simulink model "mcb_microchip_pmsm_posCtrl_SAME70"  (R2022a)
settings: Solver=FixedStepDiscrete  StartTime=0.0  StopTime=6  RelTol=1e-3  EnableMultiTasking=on
InitFcn:
  | mcb_microchip_pmsm_posCtrl_SAME70_data;
values from neighbouring files (symbols this model uses):
  PI_params = mcb.internal.SetControllerParameters(pmsm,inverter,PU_System,T_pwm,2*Ts,Ts_speed)    [mcb_microchip_pmsm_posCtrl_SAME70_data.m]
  PosCtrlSpeedLimit = 0.1    [mcb_microchip_pmsm_posCtrl_SAME70_data.m]
  PU_System = mcb_SetPUSystem(pmsm,inverter)    [mcb_microchip_pmsm_posCtrl_SAME70_data.m]
  PWM_frequency = 20e3    (= 20000)    [mcb_microchip_pmsm_posCtrl_SAME70_data.m]
  Ts = T_pwm    (= 5e-05)    [mcb_microchip_pmsm_posCtrl_SAME70_data.m]
  Ts_motor = T_pwm/2    (= 2.5e-05)    [mcb_microchip_pmsm_posCtrl_SAME70_data.m]
  Ts_simulink = T_pwm/2    (= 2.5e-05)    [mcb_microchip_pmsm_posCtrl_SAME70_data.m]
  Ts_speed = 2 * Ts    (= 0.0001)    [mcb_microchip_pmsm_posCtrl_SAME70_data.m]
undefined symbols (not defined in the file or in its folder): A24, AD10, AD7, inverter, LQFP144, MaxPer, ms, ns, PA0, PA1, PA10, PA11, PA12, PA13, PA16, PA18, PA9, PB0, PD18, PD19, PD24, PD25, PD26, Pin, pmsm, Resol, SAME70Q21B, Timer, Unsigned
libraries: MCHP_Blockset x13, simulink x13, mcbcontrolslib x8, slpidlib x3, mcbpositiondecoderlib x3, mcbplantlib x1, autolibpmsmexterior x1
(part 3 of 4)

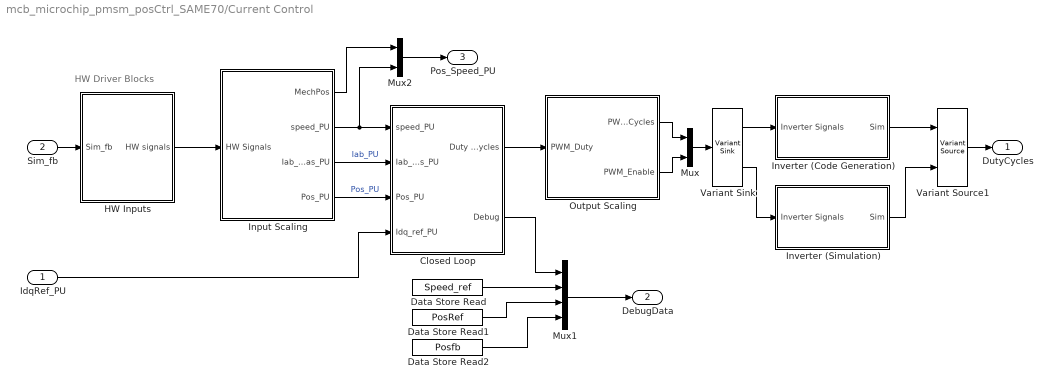
== system mcb_microchip_pmsm_posCtrl_SAME70/Current Control ==
  note: HW Driver Blocks
  IdqRef_PU : Inport
  Sim_fb : Inport  Port=2
  Closed Loop : Subsystem
  Data Store Read : DataStoreRead  DataStoreName=Speed_ref  IndexOptions=Index vector (dialog)  Indices=1  OutputSizes=1
  Data Store Read1 : DataStoreRead  DataStoreName=PosRef  IndexOptions=Index vector (dialog)  Indices=1  OutputSizes=1
  Data Store Read2 : DataStoreRead  DataStoreName=Posfb  IndexOptions=Index vector (dialog)  Indices=1  OutputSizes=1
  HW Inputs : Subsystem  Variant=on  VariantControlMode=sim codegen switching
  Input Scaling : Subsystem
  Inverter (Code Generation) : Subsystem
  Inverter (Simulation) : Subsystem
  Mux : Mux  Inputs=2
  Mux1 : Mux
  Mux2 : Mux  Inputs=2
  Output Scaling : Subsystem
  Variant Sink : VariantSink  VariantControlMode=sim codegen switching
  Variant Source1 : VariantSource  VariantControlMode=sim codegen switching
  DutyCycles : Outport  InitialOutput=0  VectorParamsAs1DForOutWhenUnconnected=off
  DebugData : Outport  Port=2
  Pos_Speed_PU : Outport  Port=3  InitialOutput=0  VectorParamsAs1DForOutWhenUnconnected=off
  wires:
  Closed Loop/1(Duty Cycles) -> Output Scaling/1(PWM_Duty)
  IdqRef_PU/1 -> Closed Loop/4(Idq_ref_PU)
  Output Scaling/2(PWM_Enable) -> Mux/2
  Input Scaling/2(speed_PU) -> Mux2/2, Closed Loop/1(speed_PU)
  Sim_fb/1 -> HW Inputs/1(Sim_fb)
  Input Scaling/3(Iab_meas_PU) -> Closed Loop/2(Iab_meas_PU)  "Iab_PU"
  Input Scaling/4(Pos_PU) -> Closed Loop/3(Pos_PU)  "Pos_PU"
  Variant Source1/1 -> DutyCycles/1
  Output Scaling/1(PWM_Duty_Cycles) -> Mux/1
  Variant Sink/2 -> Inverter (Simulation)/1(Inverter Signals)
  Inverter (Code Generation)/1(Sim) -> Variant Source1/1
  Inverter (Simulation)/1(Sim) -> Variant Source1/2
  Variant Sink/1 -> Inverter (Code Generation)/1(Inverter Signals)
  Mux/1 -> Variant Sink/1
  HW Inputs/1(HW signals) -> Input Scaling/1(HW Signals)
  Mux1/1 -> DebugData/1
  Closed Loop/2(Debug) -> Mux1/1
  Data Store Read/1 -> Mux1/2
  Mux2/1 -> Pos_Speed_PU/1
  Input Scaling/1(MechPos) -> Mux2/1
  Data Store Read1/1 -> Mux1/3
  Data Store Read2/1 -> Mux1/4

== system mcb_microchip_pmsm_posCtrl_SAME70/Heartbeat LED ==
  note: Heartbeat LED 1HZ
  Code generation : Subsystem
  RED_LED : Constant  OutDataTypeStr=uint16  SampleTime=0.25
  Simulation : Subsystem
  Variant Sink : VariantSink
  wires:
  RED_LED/1 -> Variant Sink/1
  Variant Sink/1 -> Code generation/1(In1)
  Variant Sink/2 -> Simulation/1(In1)

== system mcb_microchip_pmsm_posCtrl_SAME70/Inverter and Motor ==
  Duty_Cycles : Inport
  Plant Model : Subsystem  Variant=on  VariantControlMode=sim codegen switching  VariantControl=Variant1  PropagateVariantConditions=on
  Sim_fb : Outport  VectorParamsAs1DForOutWhenUnconnected=off
  wires:
  Duty_Cycles/1 -> Plant Model/1(Duty_Cycles)
  Plant Model/1(Sim_fb) -> Sim_fb/1

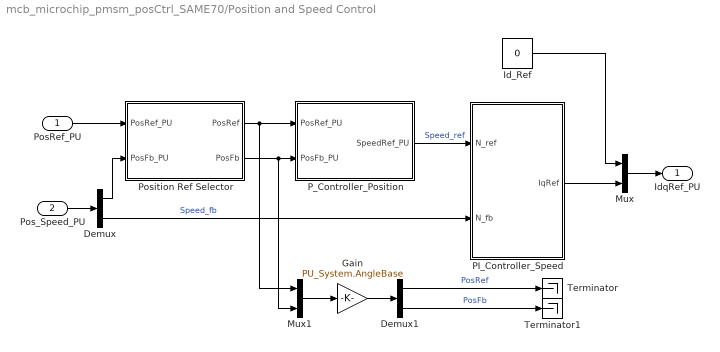
== system mcb_microchip_pmsm_posCtrl_SAME70/Position and Speed Control ==
  PosRef_PU : Inport
  Pos_Speed_PU : Inport  Port=2
  Demux : Demux  Outputs=2
  Demux1 : Demux  Outputs=2
  Gain : Gain  Gain=PU_System.AngleBase  RndMeth=Simplest  OutDataTypeStr=Inherit: Same as input
  Id_Ref : Constant  Value=0  OutDataTypeStr=dataType
  Mux : Mux  Inputs=2
  Mux1 : Mux  Inputs=2
  PI_Controller_Speed : Subsystem
  P_Controller_Position : Subsystem
  Position Ref Selector : Subsystem
  Terminator : Terminator
  Terminator1 : Terminator
  IdqRef_PU : Outport  VectorParamsAs1DForOutWhenUnconnected=off
  wires:
  Id_Ref/1 -> Mux/1
  Mux/1 -> IdqRef_PU/1
  P_Controller_Position/1(SpeedRef_PU) -> PI_Controller_Speed/1(N_ref)  "Speed_ref"
  PI_Controller_Speed/1(IqRef) -> Mux/2
  Position Ref Selector/2(PosFb) -> Mux1/2, P_Controller_Position/2(PosFb_PU)
  Position Ref Selector/1(PosRef) -> Mux1/1, P_Controller_Position/1(PosRef_PU)
  PosRef_PU/1 -> Position Ref Selector/1(PosRef_PU)
  Demux/2 -> PI_Controller_Speed/2(N_fb)  "Speed_fb"
  Pos_Speed_PU/1 -> Demux/1
  Demux/1 -> Position Ref Selector/2(PosFb_PU)
  Mux1/1 -> Gain/1
  Gain/1 -> Demux1/1
  Demux1/1 -> Terminator/1  "PosRef"
  Demux1/2 -> Terminator1/1  "PosFb"

== system mcb_microchip_pmsm_posCtrl_SAME70/Serial Receive ==
  CodeGen : Subsystem
  Data Store Write : DataStoreWrite  DataStoreName=Enable  IndexOptions=Index vector (dialog)  Indices=1  OutputSizes=1
  Data Store Write1 : DataStoreWrite  DataStoreName=PosRef  IndexOptions=Index vector (dialog)  Indices=1  OutputSizes=1
  Sim : Subsystem
  Variant Source : VariantSource  VariantControlMode=sim codegen switching
  Variant Source1 : VariantSource  VariantControlMode=sim codegen switching
  PosRef : Outport
  wires:
  Variant Source1/1 -> Data Store Write/1
  Sim/1(PosRef) -> Variant Source/2
  Sim/2(Enable) -> Variant Source1/2
  CodeGen/1(PosRef) -> Variant Source/1
  CodeGen/2(Enable) -> Variant Source1/1
  Variant Source/1 -> Data Store Write1/1, PosRef/1

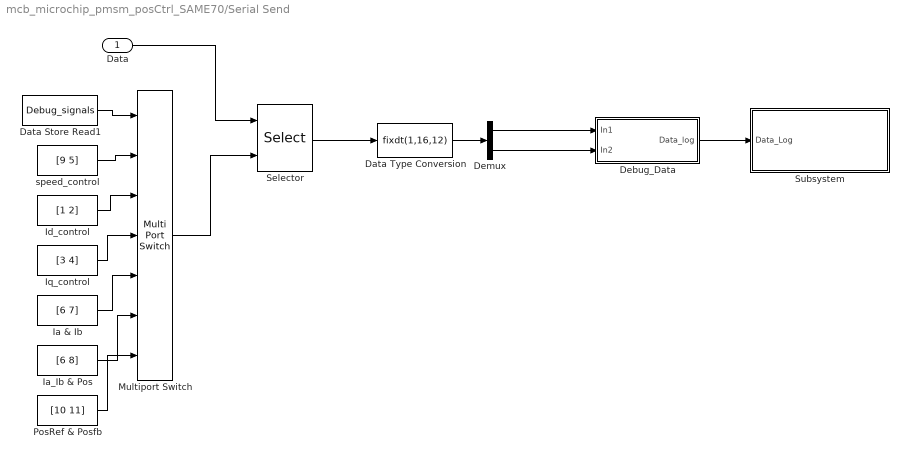
== system mcb_microchip_pmsm_posCtrl_SAME70/Serial Send ==
  Data : Inport
  Data Store Read1 : DataStoreRead  DataStoreName=Debug_signals  IndexOptions=Index vector (dialog)  Indices=1  OutputSizes=1
  Data Type Conversion : DataTypeConversion  OutDataTypeStr=fixdt(1,16,12)  RndMeth=Simplest  SaturateOnIntegerOverflow=off
  Debug_Data : Subsystem
  Demux : Demux  Outputs=2
  Ia & Ib : Constant  Value=[6 7]  OutDataTypeStr=uint16  SampleTime=-1
  Ia_Ib & Pos : Constant  Value=[6 8]  OutDataTypeStr=uint16  SampleTime=-1
  Id_control : Constant  Value=[1 2]  OutDataTypeStr=uint16  SampleTime=-1
  Iq_control : Constant  Value=[3 4]  OutDataTypeStr=uint16  SampleTime=-1
  Multiport Switch : MultiPortSwitch  Inputs=6  DiagnosticForDefault=Warning  OutDataTypeStr=uint16  RndMeth=Simplest  SaturateOnIntegerOverflow=off  InputSameDT=off
  PosRef & Posfb : Constant  Value=[10 11]  OutDataTypeStr=uint16  SampleTime=-1
  Selector : Selector  InputPortWidth=11  IndexOptions=Index vector (port)  Indices=[1 3]  OutputSizes=1
  Subsystem : Subsystem
  speed_control : Constant  Value=[9 5]  OutDataTypeStr=uint16  SampleTime=-1
  wires:
  speed_control/1 -> Multiport Switch/2
  Id_control/1 -> Multiport Switch/3
  Iq_control/1 -> Multiport Switch/4
  Ia & Ib/1 -> Multiport Switch/5
  Ia_Ib & Pos/1 -> Multiport Switch/6
  Multiport Switch/1 -> Selector/2
  Data Store Read1/1 -> Multiport Switch/1
  Debug_Data/1(Data_log) -> Subsystem/1(Data_Log)
  Data Type Conversion/1 -> Demux/1
  Demux/1 -> Debug_Data/1(In1)
  Demux/2 -> Debug_Data/2(In2)
  Data/1 -> Selector/1
  Selector/1 -> Data Type Conversion/1
  PosRef & Posfb/1 -> Multiport Switch/7

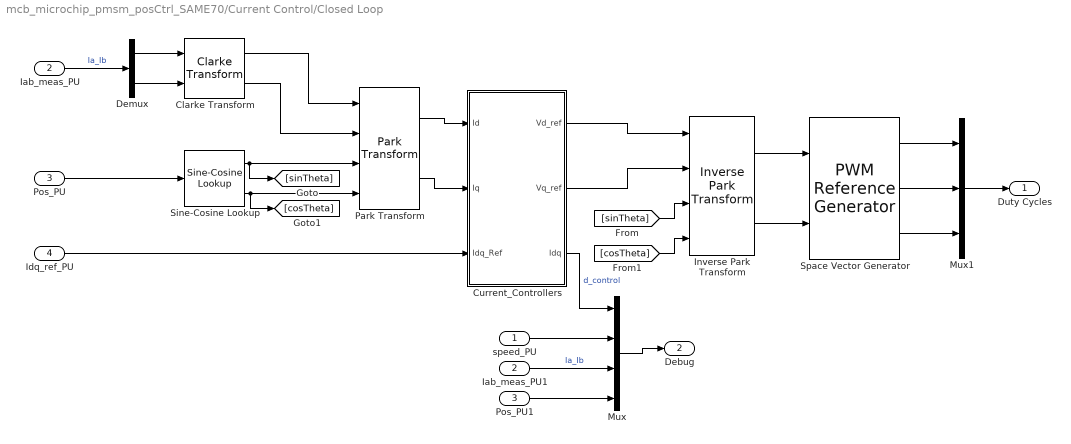
== system mcb_microchip_pmsm_posCtrl_SAME70/Current Control/Closed Loop ==
  speed_PU : Inport
  Iab_meas_PU : Inport  Port=2
  Pos_PU : Inport  Port=3
  Idq_ref_PU : Inport  Port=4
  Clarke Transform : mcbcontrolslib/Clarke Transform  VariantControl=Variant2
  Current_Controllers : Subsystem
  Demux : Demux  Outputs=2
  Iab_meas_PU1 : InportShadow  Port=2
  Inverse Park Transform : mcbcontrolslib/Inverse Park Transform  AxisAlignment=D-axis
  Mux : Mux
  Mux1 : Mux  Inputs=3
  Park Transform : mcbcontrolslib/Park Transform  AxisAlignment=D-axis
      settings: SourceProductBaseCode=MT
  Pos_PU1 : InportShadow  Port=3
  Sine-Cosine Lookup : mcbcontrolslib/Sine-Cosine Lookup  AngleInput=Per-unit  N_points=1024
      settings: SourceProductBaseCode=MT
  Space Vector Generator : mcbcontrolslib/PWM Reference Generator  inSignal=Valphabeta  modType=SVM: space vector modulation
      settings: SourceProductBaseCode=MT
  Duty Cycles : Outport  VectorParamsAs1DForOutWhenUnconnected=off
  Debug : Outport  Port=2  VectorParamsAs1DForOutWhenUnconnected=off
  wires:
  [cosTheta] -> Inverse Park Transform/4
  Inverse Park Transform/2 -> Space Vector Generator/2
  Inverse Park Transform/1 -> Space Vector Generator/1
  [sinTheta] -> Inverse Park Transform/3
  Clarke Transform/1 -> Park Transform/1
  Clarke Transform/2 -> Park Transform/2
  Sine-Cosine Lookup/1 -> [sinTheta], Park Transform/3
  Space Vector Generator/1 -> Mux1/1
  Space Vector Generator/3 -> Mux1/3
  Mux1/1 -> Duty Cycles/1
  Sine-Cosine Lookup/2 -> Park Transform/4, [cosTheta]
  Space Vector Generator/2 -> Mux1/2
  Park Transform/1 -> Current_Controllers/1(Id)
  Park Transform/2 -> Current_Controllers/2(Iq)
  Demux/1 -> Clarke Transform/1
  Demux/2 -> Clarke Transform/2
  Iab_meas_PU/1 -> Demux/1  "Ia_Ib"
  Idq_ref_PU/1 -> Current_Controllers/3(Idq_Ref)
  speed_PU/1 -> Mux/2
  Current_Controllers/3(Idq) -> Mux/1  "d_control"
  Mux/1 -> Debug/1
  Iab_meas_PU1/1 -> Mux/3  "Ia_Ib"
  Pos_PU1/1 -> Mux/4
  Pos_PU/1 -> Sine-Cosine Lookup/1
  Current_Controllers/2(Vq_ref) -> Inverse Park Transform/2
  Current_Controllers/1(Vd_ref) -> Inverse Park Transform/1

== system mcb_microchip_pmsm_posCtrl_SAME70/Current Control/HW Inputs ==
  Sim_fb : Inport
  Sensor Driver Blocks (codegen) : Subsystem  VariantControl=(codegen)
  Sensor Driver Blocks (sim) : Subsystem  VariantControl=(sim)
  HW signals : Outport

== system mcb_microchip_pmsm_posCtrl_SAME70/Current Control/Input Scaling ==
  note: Current Measurements
  HW Signals : Inport
  Calculate Phase Currents : Subsystem
  Calculate position and speed : Subsystem
  Demux : Demux  Outputs=3
  Mux : Mux  Inputs=2
  MechPos : Outport
  speed_PU : Outport  Port=2
  Iab_meas_PU : Outport  Port=3
  Pos_PU : Outport  Port=4
  wires:
  Calculate Phase Currents/1(Iab_meas_PU) -> Iab_meas_PU/1  "Iab_fb_PU"
  HW Signals/1 -> Demux/1
  Calculate position and speed/1(speed_PU) -> speed_PU/1
  Calculate position and speed/2(Pos_PU) -> Pos_PU/1
  Demux/3 -> Calculate position and speed/1(Encoder Counts)  "QDEC Counts"
  Demux/2 -> Mux/2
  Demux/1 -> Mux/1
  Mux/1 -> Calculate Phase Currents/1(Iab_ADC)  "Iab_ADC"
  Calculate position and speed/3(MechPos) -> MechPos/1

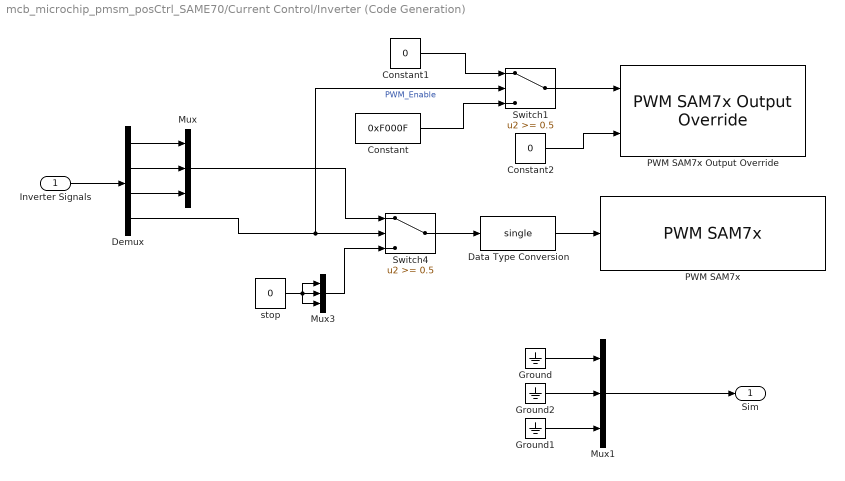
== system mcb_microchip_pmsm_posCtrl_SAME70/Current Control/Inverter (Code Generation) ==
  Inverter Signals : Inport
  Constant : Constant  Value=0xF000F  OutDataTypeStr=uint32  SampleTime=-1
  Constant1 : Constant  Value=0  OutDataTypeStr=uint32  SampleTime=-1
  Constant2 : Constant  Value=0  OutDataTypeStr=uint32  SampleTime=-1
  Data Type Conversion : DataTypeConversion  OutDataTypeStr=single  SaturateOnIntegerOverflow=off  RndMeth=Floor
  Demux : Demux
  Ground : Ground
  Ground1 : Ground
  Ground2 : Ground
  Mux : Mux  Inputs=3
  Mux1 : Mux  Inputs=3
  Mux3 : Mux  Inputs=3
  PWM SAM7x : MCHP_Blockset/PWM IO/PWM SAM7x  Priority=-2000  PWMx=PWM Controller 0  MaxPeriod_s=Ts  PWM0_pinH0=Dynamic Options  PWM0_pinH0_TXT=PA11 / Pin[64]  PWM0_pinL0=Dynamic Options  PWM0_pinL0_TXT=PD24 / Pin[55]  PWM0_pinH1=Dynamic Options  PWM0_pinH1_TXT=PA12 / Pin[68]  PWM0_pinL1=Dynamic Options  PWM0_pinL1_TXT=PD25 / Pin[52]  PWM0_pinH2=Dynamic Options  PWM0_pinH2_TXT=PA13 / Pin[42]  PWM0_pinL2=Dynamic Options  PWM0_pinL2_TXT=PD26 / Pin[53]  PWM0_pinH3=Dynamic Options  PWM0_pinH3_TXT=Not Used  PWM0_pinL3=Dynamic Options  PWM0_pinL3_TXT=Not Used  PWM1_pinH0=Dynamic Options  PWM1_pinH0_TXT=Not Used  PWM1_pinL0=Dynamic Options  PWM1_pinL0_TXT=Not Used  PWM1_pinH1=Dynamic Options  PWM1_pinH1_TXT=Not Used  PWM1_pinL1=Dynamic Options  PWM1_pinL1_TXT=Not Used  PWM1_pinH2=Dynamic Options  PWM1_pinH2_TXT=Not Used  PWM1_pinL2=Dynamic Options  PWM1_pinL2_TXT=Not Used  PWM1_pinH3=Dynamic Options  PWM1_pinH3_TXT=Not Used  PWM1_pinL3=Dynamic Options  PWM1_pinL3_TXT=Not Used  PWM_Centered=on  PWM_SyncWithPWM0=on  PushPull_Mode=off  SampleTime=Ts  S_INPUT=[-1]  S_INPUT_Size=[3]  S_OUTPUT=[]  S_OUTPUT_Size=[]  S_ListCustomDatatype=S.S_ListCustomDatatype={};  evalin_ws=PWM0max0=MCHP_Fun.Hex2num('40AD4C0000000000');PWM1max0=MCHP_Fun.Hex2num('40AD4C0000000000');PWM2max0=MCHP_Fun.Hex2num('40AD4C0000000000');  MCHP_PWMC_CLOCK_REQUEST=''  MCHP_PWMC_CLOCK_RESULT=''  MCHP_USER_INTERRUPTS=0  MCHP_PORT={PWM0H0 }{PWMH0}4:1:P11;{PWM0L0 }{PWML0}4:1:P120;{PWM0H1 }{PWMH1}4:1:P12;{PWM0L1 }{PWML1}4:1:P121;{PWM0H2 }{PWMH2}4:1:P13;{PWM0L2 }{PWML2}4:1:P122;  MCHP_MASTERLINK=mcb_microchip_pmsm_posCtrl_SAME70/Configurations/Microchip Master  invert_PWMH0=off  invert_PWML0=off  invert_PWMH1=off  invert_PWML1=off  invert_PWMH2=off  invert_PWML2=off  invert_PWMH3=off  invert_PWML3=off  InitPeriod_s=Ts  InitDutyCycle_s=0  InitDeadTimeH_s=1e-6  InitDeadTimeL_s=1e-6  InitEventLine0_ComparatorValue_s=1e-7  InitEventLine1_ComparatorValue_s=[]  BlockInput_VectorScalar=Vectors (grouped by function)  BlockInput_Period=Not a block input  BlockInput_DutyCycle=a Floating Point input within range [-1 1]  BlockInput_DeadTime=Not a block input  BlockInput_OutputOverride=Not a block input  Fault_FPV0=Not forced  Fault_FPV1=Not forced  Fault_FPV2=Not forced  Fault_FPV3=Not forced  Fault_Input0=does nothing  Fault_Input0_FFIL=off  Fault_Input1=does nothing  Fault_Input1_FFIL=off  Fault_Input2=does nothing  Fault_Input2_FFIL=on  Fault_Input3=does nothing  Fault_Input3_FFIL=off  Fault_Input4=does nothing  Fault_Input4_FFIL=on  Fault_Input5=does nothing  Fault_Input5_FFIL=on  Fault_Input6=does nothing  Fault_Input6_FFIL=on  Fault_Input7=does nothing  Fault_Input7_FFIL=on
      settings: SourceProductName=MPLAB Device Blocks for Simulink
  PWM SAM7x Output Override : MCHP_Blockset/PWM IO/PWM SAM7x  Output Override  Priority=-2000  PWMx=PWM Controller 0  SampleTime=Ts  S_INPUT=[-1]  S_INPUT_Size=[3]  S_OUTPUT=[]  S_OUTPUT_Size=[]  S_ListCustomDatatype=S.S_ListCustomDatatype={};  MCHP_MASTERLINK=mcb_microchip_pmsm_posCtrl_SAME70/Configurations/Microchip Master  Init_PWM_OS=0x0000  Init_PWM_OOV=0x0000  Input_PWM_OS=on  Input_PWM_OS_off=off  Input_PWM_OSS=off  Input_PWM_OSS_off=off  Input_PWM_OSSUPD=off  Input_PWM_OSSUPD_off=off  Input_PWM_OSC=off  Input_PWM_OSC_off=off  Input_PWM_OSCUPD=off  Input_PWM_OSCUPD_off=off  Input_PWM_OOV=on
      settings: SourceProductName=MPLAB Device Blocks for Simulink
  Switch1 : Switch  Threshold=0.5  RndMeth=Simplest  SaturateOnIntegerOverflow=off  InputSameDT=off
  Switch4 : Switch  Threshold=0.5  RndMeth=Simplest  SaturateOnIntegerOverflow=off  InputSameDT=off
  stop : Constant  Value=0  OutDataTypeStr=dataType
  Sim : Outport  VectorParamsAs1DForOutWhenUnconnected=off
  wires:
  Inverter Signals/1 -> Demux/1
  Ground/1 -> Mux1/1
  Ground1/1 -> Mux1/3
  Ground2/1 -> Mux1/2
  Mux1/1 -> Sim/1
  Demux/1 -> Mux/1
  Demux/2 -> Mux/2
  Demux/3 -> Mux/3
  Switch4/1 -> Data Type Conversion/1
  Data Type Conversion/1 -> PWM SAM7x/1
  stop/1 -> Mux3/3, Mux3/2, Mux3/1
  Mux/1 -> Switch4/1
  Mux3/1 -> Switch4/3
  Demux/4 -> Switch1/2, Switch4/2  "PWM_Enable"
  Switch1/1 -> PWM SAM7x Output Override/1
  Constant1/1 -> Switch1/1
  Constant/1 -> Switch1/3
  Constant2/1 -> PWM SAM7x Output Override/2

== system mcb_microchip_pmsm_posCtrl_SAME70/Current Control/Inverter (Simulation) ==
  Inverter Signals : Inport
  Data Type Duplicate : DataTypeDuplicate
  Demux : Demux
  Mux : Mux  Inputs=3
  Mux2 : Mux  Inputs=3
  Subsystem : Subsystem
  Switch1 : Switch  Threshold=0.5  RndMeth=Simplest  SaturateOnIntegerOverflow=off  InputSameDT=off
  stop : Constant  Value=0  OutDataTypeStr=Inherit: Inherit via back propagation
  Sim : Outport  VectorParamsAs1DForOutWhenUnconnected=off
  wires:
  stop/1 -> Data Type Duplicate/2, Mux2/1, Mux2/3, Mux2/2
  Mux2/1 -> Switch1/3
  Switch1/1 -> Sim/1
  Inverter Signals/1 -> Demux/1
  Demux/4 -> Switch1/2  "PWM Enable"
  Mux/1 -> Subsystem/1(In1), Data Type Duplicate/1  "PWM Duty Cycles"
  Demux/1 -> Mux/1
  Demux/2 -> Mux/2
  Demux/3 -> Mux/3
  Subsystem/1(PWM_Duty_Cycles) -> Switch1/1

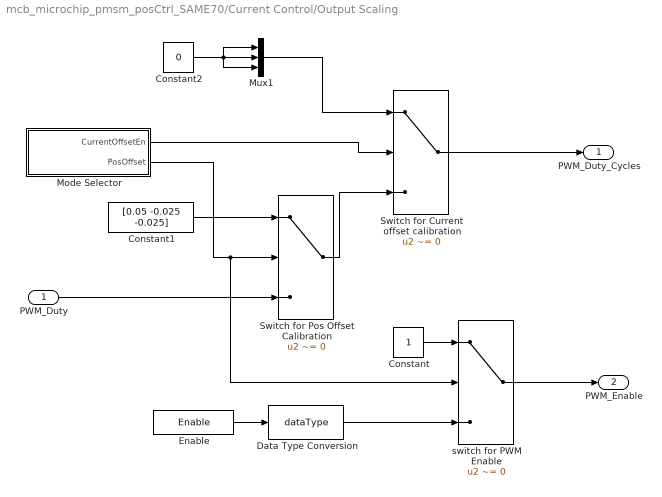
== system mcb_microchip_pmsm_posCtrl_SAME70/Current Control/Output Scaling ==
  PWM_Duty : Inport
  Constant : Constant  OutDataTypeStr=dataType
  Constant1 : Constant  Value=[0.05 -0.025 -0.025]  OutDataTypeStr=Inherit: Inherit via back propagation
  Constant2 : Constant  Value=0  OutDataTypeStr=Inherit: Inherit via back propagation
  Data Type Conversion : DataTypeConversion  OutDataTypeStr=dataType  SaturateOnIntegerOverflow=off  RndMeth=Floor
  Enable : DataStoreRead  DataStoreName=Enable  IndexOptions=Index vector (dialog)  Indices=1  OutputSizes=1
  Mode Selector : Subsystem
  Mux1 : Mux  Inputs=3
  Switch for Current offset calibration : Switch  Criteria=u2 ~= 0  Threshold=250  SaturateOnIntegerOverflow=off  InputSameDT=off
  Switch for Pos Offset Calibration : Switch  Criteria=u2 ~= 0  Threshold=250  SaturateOnIntegerOverflow=off  InputSameDT=off
  switch for PWM Enable : Switch  Criteria=u2 ~= 0  Threshold=250  SaturateOnIntegerOverflow=off  InputSameDT=off
  PWM_Duty_Cycles : Outport
  PWM_Enable : Outport  Port=2
  wires:
  Enable/1 -> Data Type Conversion/1
  Mode Selector/1(CurrentOffsetEn) -> Switch for Current offset calibration/2
  Mux1/1 -> Switch for Current offset calibration/1
  Constant2/1 -> Mux1/3, Mux1/2, Mux1/1
  Switch for Current offset calibration/1 -> PWM_Duty_Cycles/1
  Switch for Pos Offset Calibration/1 -> Switch for Current offset calibration/3
  Mode Selector/2(PosOffset) -> Switch for Pos Offset Calibration/2, switch for PWM Enable/2
  Constant1/1 -> Switch for Pos Offset Calibration/1
  PWM_Duty/1 -> Switch for Pos Offset Calibration/3
  switch for PWM Enable/1 -> PWM_Enable/1
  Data Type Conversion/1 -> switch for PWM Enable/3
  Constant/1 -> switch for PWM Enable/1

== system mcb_microchip_pmsm_posCtrl_SAME70/Heartbeat LED/Code generation ==
  In1 : Inport
  DBG LED 1 : MCHP_Blockset/Digital IO/Digital Output Write  PORT=Dynamic Options  PORT_TXT="C   [ 0 : 31 ]"  PIN=23  PACK=off  SIMULTANEOUS=off  ORDERING=None  SampleTime=-1  MCHP_PORT={Digital Out}{DOU}1:1:C23;  MCHP_MASTERLINK=mcb_microchip_pmsm_posCtrl_SAME70/Configurations/Microchip Master
      settings: SourceProductName=MPLAB Device Blocks for Simulink
  Delay 10Hz : Delay  DelayLength=1  InitialCondition=0  SampleTime=0.25
  Logical Operator : Logic  Operator=NOT  AllPortsSameDT=off  OutDataTypeStr=boolean
  Terminator : Terminator
  wires:
  Logical Operator/1 -> DBG LED 1/1, Delay 10Hz/1
  Delay 10Hz/1 -> Logical Operator/1
  In1/1 -> Terminator/1

== system mcb_microchip_pmsm_posCtrl_SAME70/Heartbeat LED/Simulation ==
  In1 : Inport
  Simulation_Terminator : Terminator
  wires:
  In1/1 -> Simulation_Terminator/1

== system mcb_microchip_pmsm_posCtrl_SAME70/Inverter and Motor/Plant Model ==
  Duty_Cycles : Inport
  Inverter and Motor (codegen) : Subsystem  VariantControl=(codegen)
  Inverter and Motor (sim) : Subsystem  VariantControl=(sim)
  Sim_fb : Outport  VectorParamsAs1DForOutWhenUnconnected=off

== system mcb_microchip_pmsm_posCtrl_SAME70/Position and Speed Control/PI_Controller_Speed ==
  N_ref : Inport
  N_fb : Inport  Port=2
  AND : Logic  IconShape=distinctive  AllPortsSameDT=off  OutDataTypeStr=boolean
  Data Store Read2 : DataStoreRead  DataStoreName=EnClosedLoop  IndexOptions=Index vector (dialog)  Indices=1  OutputSizes=1
  Data Store Read1 : DataStoreRead  DataStoreName=Enable  IndexOptions=Index vector (dialog)  Indices=1  OutputSizes=1
  Discrete PI Controller with anti-windup & reset : slpidlib/PID Controller  Controller=PI  Form=Parallel  TimeDomain=Discrete-time  UseExternalTs=off  SampleTime=-1  IntegratorMethod=Forward Euler  FilterMethod=Forward Euler  ControllerParametersSource=external  P=1  I=1  UseKiTs=on  D=0  N=100  UseFilter=on  TunerSelectOption=Transfer Function Based (PID Tuner App)  InitialConditionSource=external  InitialConditionForIntegrator=0  InitialConditionForFilter=0  DifferentiatorICPrevScaledInput=0  ExternalReset=level  TrackingMode=off  Kt=1  LimitOutput=on  SatLimitsSource=internal  UpperSaturationLimit=1  LowerSaturationLimit=-1  LinearizeAsGain=on  AntiWindupMode=clamping  Kb=1  RndMeth=Simplest  POutMin=[]  POutMax=[]  IOutMin=[]  IOutMax=[]  DOutMin=[]  DOutMax=[]  NOutMin=[]  NOutMax=[]  SumOutMin=[]  SumOutMax=[]  SaturationOutDataTypeStr=Inherit: Inherit via back propagation  SaturationOutMin=[]  SaturationOutMax=[]  PParamMin=[]  PParamMax=[]  IParamMin=[]  IParamMax=[]  DParamMin=[]  DParamMax=[]  NParamMin=[]  NParamMax=[]  KbParamMin=[]  KbParamMax=[]  KtParamMin=[]  KtParamMax=[]  KbOutMin=[]  KbOutMax=[]  KtOutMin=[]  KtOutMax=[]  IntegratorOutMin=[]  IntegratorOutMax=[]  FilterOutMin=[]  FilterOutMax=[]  SumI1OutMin=[]  SumI1OutMax=[]  SumI2OutMin=[]  SumI2OutMax=[]  SumI3OutMin=[]  SumI3OutMax=[]  SumI4OutMin=[]  SumI4OutMax=[]  SumDOutMin=[]  SumDOutMax=[]  DifferentiatorOutMin=[]  DifferentiatorOutMax=[]  FilterDiffOutCoefMin=[]  FilterDiffOutCoefMax=[]  ReciprocalOutMin=[]  ReciprocalOutMax=[]  SumDenOutMin=[]  SumDenOutMax=[]  SumNumOutMin=[]  SumNumOutMax=[]  DivideOutMin=[]  DivideOutMax=[]  UdiffTsProdOutMin=[]  UdiffTsProdOutMax=[]  NTsProdOutMin=[]  NTsProdOutMax=[]  UintegralTsProdOutMin=[]  UintegralTsProdOutMax=[]  UngainTsProdOutMin=[]  UngainTsProdOutMax=[]  IntegratorContinuousStateAttributes=''  IntegratorStateMustResolveToSignalObject=off  IntegratorRTWStateStorageClass=Auto  FilterContinuousStateAttributes=''  FilterStateMustResolveToSignalObject=off  FilterRTWStateStorageClass=Auto  ParallelPVariant=ExternalParameters  IdealPVariant=Disabled  IVariant=ExternalParameters  DVariant=Disabled  IntegratorVariant=Discrete  SatVariant=Enabled  AWVariant=DiscClampingParallel  PCopyVariant=Disabled  TRVariant=Disabled  FdbkBlocksVariant=Forward  IdealPFdbkVariant=Disabled  SatFdbkVariant=Disabled  DerivativeFilterVariant=Disabled  NVariant=Disabled  NCopyVariant=Disabled_SignalSpec  FilterICVariant=Disabled  IntegratorICVariant=ExternalICs  ExternalResetVariant=ExternalReset  TRSumVariant=Passthrough  SumFdbkVariant=Disabled  SumVariant=Sum_PI  TsampFilterVariant=InternalTs  TsampNgainVariant=Passthrough  TsampIntegralVariant=Passthrough  ExternalSaturationOutDataTypeStr=Inherit: Same as second input  aMode=5
      settings: SourceProductBaseCode=MT
  Ki1 : Constant  Value=PI_params.Ki_speed*Ts_speed  OutDataTypeStr=dataType  SampleTime=-1
  Ki2 : Constant  Value=0  OutDataTypeStr=dataType  SampleTime=-1
  Kp1 : Constant  Value=PI_params.Kp_speed  OutDataTypeStr=dataType  SampleTime=-1
  Logical Operator : Logic  Operator=NOT  IconShape=distinctive  AllPortsSameDT=off  OutDataTypeStr=boolean
  Sum : Sum  Inputs=|+-  OutDataTypeStr=Inherit: Same as first input
  IqRef : Outport  VectorParamsAs1DForOutWhenUnconnected=off
  wires:
  Discrete PI Controller with anti-windup & reset/1 -> IqRef/1
  Ki1/1 -> Discrete PI Controller with anti-windup & reset/3
  Kp1/1 -> Discrete PI Controller with anti-windup & reset/2
  N_fb/1 -> Sum/2
  N_ref/1 -> Sum/1
  Sum/1 -> Discrete PI Controller with anti-windup & reset/1
  Logical Operator/1 -> Discrete PI Controller with anti-windup & reset/4
  Ki2/1 -> Discrete PI Controller with anti-windup & reset/5
  Data Store Read1/1 -> AND/1
  Data Store Read2/1 -> AND/2
  AND/1 -> Logical Operator/1

== system mcb_microchip_pmsm_posCtrl_SAME70/Position and Speed Control/P_Controller_Position ==
  PosRef_PU : Inport
  PosFb_PU : Inport  Port=2
  Constant : Constant  Value=PI_params.Kp_PosCtrl  OutDataTypeStr=dataType
  Data Store Write3 : DataStoreWrite  DataStoreName=Speed_ref  IndexOptions=Index vector (dialog)  Indices=1  OutputSizes=1
  Divide : Product  Inputs=**  OutDataTypeStr=dataType  RndMeth=Simplest
  Saturation : Saturate  UpperLimit=PosCtrlSpeedLimit  LowerLimit=-PosCtrlSpeedLimit
  Sum : Sum  Inputs=|+-  OutDataTypeStr=Inherit: Same as first input
  SpeedRef_PU : Outport
  wires:
  Sum/1 -> Divide/1
  PosFb_PU/1 -> Sum/2
  PosRef_PU/1 -> Sum/1
  Divide/1 -> Saturation/1
  Constant/1 -> Divide/2
  Saturation/1 -> SpeedRef_PU/1, Data Store Write3/1

== system mcb_microchip_pmsm_posCtrl_SAME70/Position and Speed Control/Position Ref Selector ==
  PosRef_PU : Inport
  PosFb_PU : Inport  Port=2
  AND : Logic  IconShape=distinctive  AllPortsSameDT=off  OutDataTypeStr=boolean
  Data Store Read : DataStoreRead  DataStoreName=EnClosedLoop  IndexOptions=Index vector (dialog)  Indices=1  OutputSizes=1
  Data Store Write1 : DataStoreWrite  DataStoreName=Posfb  IndexOptions=Index vector (dialog)  Indices=1  OutputSizes=1
  Data Store Read1 : DataStoreRead  DataStoreName=Enable  IndexOptions=Index vector (dialog)  Indices=1  OutputSizes=1
  Switch : Switch  Criteria=u2 > Threshold  SaturateOnIntegerOverflow=off  InputSameDT=off
  PosRef : Outport
  PosFb : Outport  Port=2
  wires:
  PosFb_PU/1 -> Switch/3, PosFb/1, Data Store Write1/1
  Switch/1 -> PosRef/1
  Data Store Read1/1 -> AND/2
  PosRef_PU/1 -> Switch/1
  AND/1 -> Switch/2
  Data Store Read/1 -> AND/1

== system mcb_microchip_pmsm_posCtrl_SAME70/Serial Receive/CodeGen ==
  Data Store Write1 : DataStoreWrite  DataStoreName=Debug_signals  IndexOptions=Index vector (dialog)  Indices=1  OutputSizes=1
  Data Type Conversion : DataTypeConversion  OutDataTypeStr=uint16  SaturateOnIntegerOverflow=off  RndMeth=Floor
  Subsystem : Subsystem
  Subsystem1 : Subsystem
  UART Rx : MCHP_Blockset/BUS UART/UART Rx  UART_REF=UART 0  Flag_Out=on  Rx_Size_popup=User defined  Rx_Size=1  S_Rx_Size=1  Split=Read all received char  SplitChar=10  OutputDefault_popup=do nothing (end of output vector will be undefined)  OutputDefault=-2  ORDERING=None  SampleTime=.001  MCHP_MASTERLINK=mcb_microchip_pmsm_posCtrl_SAME70/Configurations/Microchip Master  MCHP_COMPILED_INFO="CompiledSampleTime= [0.0010000000000000000208   0 ];CompiledInportDataTypes=[    ];CompiledInportDataWidth=[];"
      settings: SourceProductName=MPLAB Device Blocks for Simulink
  PosRef : Outport
  Enable : Outport  Port=2
  wires:
  UART Rx/1 -> Data Type Conversion/1
  Subsystem/3(Debug Signal Selection) -> Data Store Write1/1
  UART Rx/2 -> Subsystem1/1(In1)
  Subsystem/2(Enable) -> Enable/1
  Subsystem/1(PosRef) -> PosRef/1
  Subsystem1/2(Data out) -> Subsystem/1(In1)
  Subsystem1/1(NewData) -> Subsystem/Enable
  Data Type Conversion/1 -> Subsystem1/Enable

== system mcb_microchip_pmsm_posCtrl_SAME70/Serial Receive/Sim ==
  Data Type Conversion1 : DataTypeConversion  OutDataTypeStr=dataType  RndMeth=Simplest  SaturateOnIntegerOverflow=off
  Data Type Conversion2 : DataTypeConversion  OutDataTypeStr=boolean  RndMeth=Simplest  SaturateOnIntegerOverflow=off
  Gain : Gain  Gain=1/PU_System.AngleBase  RndMeth=Simplest  OutDataTypeStr=Inherit: Same as input
  Pos Ref [Degrees] : Step  Time=3.5  Before=500  After=-653  OutDataTypeStr=single  SampleTime=0.001
  Step1 : Step  OutDataTypeStr=single  SampleTime=0.001
  PosRef : Outport
  Enable : Outport  Port=2
  wires:
  Pos Ref [Degrees]/1 -> Gain/1
  Data Type Conversion1/1 -> PosRef/1
  Step1/1 -> Data Type Conversion2/1
  Data Type Conversion2/1 -> Enable/1
  Gain/1 -> Data Type Conversion1/1

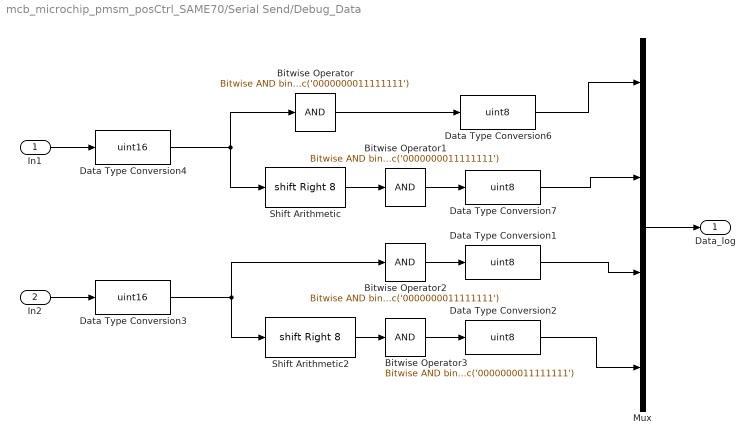
== system mcb_microchip_pmsm_posCtrl_SAME70/Serial Send/Debug_Data ==
  In1 : Inport
  In2 : Inport  Port=2
  Bitwise Operator{,1..3} (4 alike) : simulink/Logic and Bit Operations/Bitwise Operator  logicop=AND  UseBitMask=on  BitMask=bin2dec('0000000011111111')  BitMaskRealWorld=Stored Integer
  Data Type Conversion{1..2,6..7} (4 alike) : DataTypeConversion  OutDataTypeStr=uint8  RndMeth=Simplest  SaturateOnIntegerOverflow=off
  Data Type Conversion3 : DataTypeConversion  OutDataTypeStr=uint16  ConvertRealWorld=Stored Integer (SI)  RndMeth=Simplest  SaturateOnIntegerOverflow=off
  Data Type Conversion4 : DataTypeConversion  OutDataTypeStr=uint16  ConvertRealWorld=Stored Integer (SI)  RndMeth=Simplest  SaturateOnIntegerOverflow=off
  Mux : Mux
  Shift Arithmetic : ArithShift  BitShiftNumber=8  BitShiftDirection=Right
  Shift Arithmetic2 : ArithShift  BitShiftNumber=8  BitShiftDirection=Right
  Data_log : Outport
  wires:
  Mux/1 -> Data_log/1
  In1/1 -> Data Type Conversion4/1
  Data Type Conversion4/1 -> Shift Arithmetic/1, Bitwise Operator/1
  Data Type Conversion6/1 -> Mux/1
  Data Type Conversion7/1 -> Mux/2
  Bitwise Operator2/1 -> Data Type Conversion1/1
  Data Type Conversion1/1 -> Mux/3
  Bitwise Operator/1 -> Data Type Conversion6/1
  Shift Arithmetic/1 -> Bitwise Operator1/1
  Data Type Conversion2/1 -> Mux/4
  Bitwise Operator1/1 -> Data Type Conversion7/1
  Shift Arithmetic2/1 -> Bitwise Operator3/1
  Bitwise Operator3/1 -> Data Type Conversion2/1
  Data Type Conversion3/1 -> Shift Arithmetic2/1, Bitwise Operator2/1
  In2/1 -> Data Type Conversion3/1

== system mcb_microchip_pmsm_posCtrl_SAME70/Serial Send/Subsystem ==
  note: Fast Serial Data Monitoring (32-bit)
  Data_Log : Inport
  Counter Limited : simulink/Sources/Counter Limited  uplimit=119  tsamp=-1
  Data : Subsystem  TreatAsAtomicUnit=on
  End : Subsystem  TreatAsAtomicUnit=on
  If : If  IfExpression=u1 == 0  ElseIfExpressions=u1 == 119
  Start : Subsystem  TreatAsAtomicUnit=on
  wires:
  Data_Log/1 -> Data/1(Data), Start/1(Data), End/1(Data)
  If/1 -> Start/Action
  If/2 -> End/Action
  Counter Limited/1 -> If/1
  If/3 -> Data/Action

== system mcb_microchip_pmsm_posCtrl_SAME70/Current Control/Closed Loop/Current_Controllers ==
  Id : Inport
  Iq : Inport  Port=2
  Idq_Ref : Inport  Port=3
  DQ Limiter : mcbcontrolslib/DQ Limiter  Vmax=0.95
      settings: SourceProductBaseCode=MT
  Demux : Demux  Outputs=2
  Mux : Mux
  PI_Controller_Id : Subsystem
  PI_Controller_Iq : Subsystem
  Terminator : Terminator
  Vd_ref : Outport  VectorParamsAs1DForOutWhenUnconnected=off
  Vq_ref : Outport  Port=2  VectorParamsAs1DForOutWhenUnconnected=off
  Idq : Outport  Port=3  VectorParamsAs1DForOutWhenUnconnected=off
  wires:
  Iq/1 -> Mux/4, PI_Controller_Iq/2(I_fb)  "Iq_fb"
  PI_Controller_Id/1(V_ref) -> DQ Limiter/1
  Id/1 -> PI_Controller_Id/2(I_fb), Mux/2  "Id_fb"
  Demux/1 -> PI_Controller_Id/1(I_ref), Mux/1  "Id_Ref"
  Demux/2 -> Mux/3, PI_Controller_Iq/1(I_ref)  "Iq_Ref"
  DQ Limiter/1 -> Vd_ref/1
  DQ Limiter/2 -> Vq_ref/1
  PI_Controller_Iq/1(V_ref) -> DQ Limiter/2
  DQ Limiter/3 -> Terminator/1
  Idq_Ref/1 -> Demux/1
  Mux/1 -> Idq/1

== system mcb_microchip_pmsm_posCtrl_SAME70/Current Control/HW Inputs/Sensor Driver Blocks (codegen) ==
  Sim_fb : Inport
  ADC SAMx1 : MCHP_Blockset/Analog IO/ADC SAMx7  Priority=-2000  AFECx=AFE Controller 0  SIGNMODE_SingleEnded=Unsigned (uint16)  SIGNMODE_Differential=Unsigned (uint16)  AFEC0_seq0=Dynamic Options  AFEC0_seq0_TXT="AD0 / PD30   &   AD6 / PA17"  AFEC1_seq0=Dynamic Options  AFEC1_seq0_TXT=Not used  AFEC0_seq1=Dynamic Options  AFEC0_seq1_TXT=AD7 / PA18  AFEC1_seq1=Dynamic Options  AFEC1_seq1_TXT=Not used  AFEC0_seq2=Dynamic Options  AFEC0_seq2_TXT=AD10 / PB0  AFEC1_seq2=Dynamic Options  AFEC1_seq2_TXT=Not used  AFEC0_seq3=Dynamic Options  AFEC0_seq3_TXT=Not used  AFEC1_seq3=Dynamic Options  AFEC1_seq3_TXT=Not used  AFEC0_seq4=Dynamic Options  AFEC0_seq4_TXT=Not used  AFEC1_seq4=Dynamic Options  AFEC1_seq4_TXT=Not used  AFEC0_seq5=Dynamic Options  AFEC0_seq5_TXT=Not used  AFEC1_seq5=Dynamic Options  AFEC1_seq5_TXT=Not used  AFEC0_seq6=Dynamic Options  AFEC0_seq6_TXT=Not used  AFEC1_seq6=Dynamic Options  AFEC1_seq6_TXT=Not used  AFEC0_seq7=Dynamic Options  AFEC0_seq7_TXT=Not used  AFEC1_seq7=Dynamic Options  AFEC1_seq7_TXT=Not used  AFEC0_seq8=Dynamic Options  AFEC0_seq8_TXT=Not used  AFEC1_seq8=Dynamic Options  AFEC1_seq8_TXT=Not used  AFEC0_seq9=Dynamic Options  AFEC0_seq9_TXT=Not used  AFEC1_seq9=Dynamic Options  AFEC1_seq9_TXT=Not used  AFEC0_seq10=Dynamic Options  AFEC0_seq10_TXT=Not used  AFEC1_seq10=Dynamic Options  AFEC1_seq10_TXT=Not used  AFEC0_seq11=Dynamic Options  AFEC0_seq11_TXT=Not used  AFEC1_seq11=Dynamic Options  AFEC1_seq11_TXT=Not used  SampleTime=Ts  S_INPUT=[-1]  S_INPUT_Size=[3]  S_OUTPUT=[]  S_OUTPUT_Size=[]  S_ListCustomDatatype=S.S_ListCustomDatatype={};  MCHP_AFECC_CLOCK_REQUEST=''  MCHP_AFECC_CLOCK_RESULT=''  MCHP_USER_INTERRUPTS=0  MCHP_PORT={AD0 AFEC0}{AD0}15:2:P126;{AD6 AFEC0}{AD6}15:2:P17;{AD7 AFEC0}{AD7}15:2:P18;{AD10 AFEC0}{AD10}15:2:P32;  MCHP_MASTERLINK=mcb_microchip_pmsm_posCtrl_SAME70/Configurations/Microchip Master  Rin=< 200 Ohm  RES=12-bit Standard  AFEC0_Synchronisation=Triggered by user defined source  AFEC0_Trig=PWM0 event line 0  AFEC0_TrigTimeStep=on  AFEC1_Synchronisation=Triggered by user defined source  AFEC1_Trig=PWM1 event line 0  AFEC1_TrigTimeStep=off  ADC_TrigInfo=0  AFEC0_seq0_GAIN=1  AFEC1_seq0_GAIN=1  AFEC0_seq1_GAIN=1  AFEC1_seq1_GAIN=1  AFEC0_seq2_GAIN=1  AFEC1_seq2_GAIN=1  AFEC0_seq3_GAIN=1  AFEC1_seq3_GAIN=1  AFEC0_seq4_GAIN=1  AFEC1_seq4_GAIN=1  AFEC0_seq5_GAIN=1  AFEC1_seq5_GAIN=1  AFEC0_seq6_GAIN=1  AFEC1_seq6_GAIN=1  AFEC0_seq7_GAIN=1  AFEC1_seq7_GAIN=1  AFEC0_seq8_GAIN=1  AFEC1_seq8_GAIN=1  AFEC0_seq9_GAIN=1  AFEC1_seq9_GAIN=1  AFEC0_seq10_GAIN=1  AFEC1_seq10_GAIN=1  AFEC0_seq11_GAIN=1  AFEC1_seq11_GAIN=1  AFEC0_seq0_OFFSET=0  AFEC1_seq0_OFFSET=0  AFEC0_seq1_OFFSET=0  AFEC1_seq1_OFFSET=0  AFEC0_seq2_OFFSET=0  AFEC1_seq2_OFFSET=0  AFEC0_seq3_OFFSET=0  AFEC1_seq3_OFFSET=0  AFEC0_seq4_OFFSET=0  AFEC1_seq4_OFFSET=0  AFEC0_seq5_OFFSET=0  AFEC1_seq5_OFFSET=0  AFEC0_seq6_OFFSET=0  AFEC1_seq6_OFFSET=0  AFEC0_seq7_OFFSET=0  AFEC1_seq7_OFFSET=0  AFEC0_seq8_OFFSET=0  AFEC1_seq8_OFFSET=0  AFEC0_seq9_OFFSET=0  AFEC1_seq9_OFFSET=0  AFEC0_seq10_OFFSET=0  AFEC1_seq10_OFFSET=0  AFEC0_seq11_OFFSET=0  AFEC1_seq11_OFFSET=0
      settings: SourceProductName=MPLAB Device Blocks for Simulink
  Data Store Read : DataStoreRead  DataStoreName=EnPosOffset  IndexOptions=Index vector (dialog)  Indices=1  OutputSizes=1
  Mux : Mux  Inputs=3
  QDEC : MCHP_Blockset/QEI/QDEC  QDEC_REF=Dynamic Options  QDEC_REF_TXT=TC0  PHA_PIN=Dynamic Options  PHA_PIN_TXT=PA0 / Pin[102]  PHB_PIN=Dynamic Options  PHB_PIN_TXT=PA1 / Pin[99]  IDX_PIN=Dynamic Options  IDX_PIN_TXT=PA16 / Pin[45]  INVERT_PHA=off  INVERT_PHB=off  INVERT_IDX=off  SWAP_PHA_PHB=off  SampleTime=Ts  MCHP_PORT={TC0}{TIOA0}3:0:P0;{TC0}{TIOB0}3:0:P1;{TC0}{TIOB1}3:0:P16;  MCHP_MASTERLINK=mcb_microchip_pmsm_posCtrl_SAME70/Configurations/Microchip Master  MCHP_TIMER_REQUEST={Quadrature Decoder (Phase Counter)}{QDEC0}20:4:4:0:[1]:65535;{Quadrature Decoder (IDX Counter)}{QDEC0}20:4:4:0:[2]:65535;{Quadrature Decoder (Speed Measurement Time Base)}{QDEC0}20:4:4:0:[3]:65535;  MCHP_TIMER_RESULT=[1 65535]  QDEC_MODE=Position  POSITION_OUTPUT=is a 16 bits unsigned block output  INDEX_OUTPUT=is not a block output  RESET_INPUT=off  POSITION_RESET_MODE=never reset position  RESET_EDGE=rising edge  POSITION_RESET_VALUE=65535  SPEED_TIME_BASE=Dynamic Options  SPEED_TIME_BASE_TXT=Resol: 53.33(ns) - MaxPer: 3.5(ms)  SPEED_OUTPUT=is a 16 bits unsigned block output  DIR_OUTPUT=is not a block output  DIRCHG_OUTPUT=is not a block output  AUTO_CORRECTION=off  MAX_PERIOD_FILTER=Dynamic Options  MAX_PERIOD_FILTER_TXT=420(ns)  MAXCMP=disabled  MPE_OUTPUT=is not a block output  QERR_OUTPUT=is not a block output
      settings: SourceProductName=MPLAB Device Blocks for Simulink
  Qdec_interface : Subsystem  mask{EnCountPerRev=pmsm.QEPSlits*4}
      mask prompts: EnCountPerRev "Encoder counts per rev"
  Terminator : Terminator
  Terminator1 : Terminator
  Terminator2 : Terminator
  HW signals : Outport
  wires:
  Sim_fb/1 -> Terminator/1
  Mux/1 -> HW signals/1
  ADC SAMx1/4 -> Terminator2/1
  ADC SAMx1/3 -> Terminator1/1
  ADC SAMx1/1 -> Mux/1
  ADC SAMx1/2 -> Mux/2
  Data Store Read/1 -> Qdec_interface/2(Qdec_reset)
  QDEC/1 -> Qdec_interface/1(Qdec count)
  Qdec_interface/1(QDEC_Out) -> Mux/3

== system mcb_microchip_pmsm_posCtrl_SAME70/Current Control/HW Inputs/Sensor Driver Blocks (sim) ==
  Sim_fb : Inport
  HW signals : Outport
  wires:
  Sim_fb/1 -> HW signals/1

== system mcb_microchip_pmsm_posCtrl_SAME70/Current Control/Input Scaling/Calculate Phase Currents ==
  Iab_ADC : Inport
  Add : Sum  Inputs=+-
  Data Store Read2 : DataStoreRead  DataStoreName=EnCurOffset  IndexOptions=Index vector (dialog)  Indices=1  OutputSizes=1
  Data Type Conversion : DataTypeConversion  OutDataTypeStr=int32  ConvertRealWorld=Stored Integer (SI)  SaturateOnIntegerOverflow=off  RndMeth=Floor
  Data Type Conversion1 : DataTypeConversion  OutDataTypeStr=dataType  SaturateOnIntegerOverflow=off  RndMeth=Floor
  Gain1 : Gain  Gain=1/2048  OutDataTypeStr=Inherit: Same as input  ParamDataTypeStr=Inherit: Same as input
  Offset : Subsystem
  Iab_meas_PU : Outport  VectorParamsAs1DForOutWhenUnconnected=off
  wires:
  Add/1 -> Data Type Conversion1/1
  Iab_ADC/1 -> Data Type Conversion/1
  Gain1/1 -> Iab_meas_PU/1
  Data Type Conversion1/1 -> Gain1/1
  Data Store Read2/1 -> Offset/Enable
  Data Type Conversion/1 -> Add/1, Offset/1(Iab)
  Offset/1(Offset) -> Add/2

== system mcb_microchip_pmsm_posCtrl_SAME70/Current Control/Input Scaling/Calculate position and speed ==
  Encoder Counts : Inport
  Calculate Position : Subsystem
  IIR Filter4 : mcbcontrolslib/IIR Filter  VariantControl=Low Pass Filter  VariantSelect=Low-pass  Filter_constant=0.01  advancedSettings=off  Ts=50e-6  cutOff_freq=32.1525
      settings: SourceProductBaseCode=MT
  Mechanical to Electrical Position : mcbpositiondecoderlib/Mechanical to Electrical Position  NrPP=pmsm.p  selectedRange=Per unit  MechOfstInputType=Specify via dialog  mechOffsetIn=0  maxAngleIn=1  InputDataType=dataType  VariantSelect=floating-point
      settings: SourceProductBaseCode=MT
  Quadrature Decoder : mcbpositiondecoderlib/Quadrature Decoder  EncoderSlitsPerRevolution=pmsm.QEPSlits  EncoderCountsPerSlit=4  CounterSize=16 bits  ExternalIndexCount=off  PositionUnit=Per unit  PositionDataType=dataType
      settings: SourceProductBaseCode=MT
  Speed Measurement : mcbpositiondecoderlib/Speed Measurement  PositionUnit=Per unit  PositionScalingDatatype=uint32  SpeedCalculationMode=Time interval for speed calculation  SampleTimeAsync=Ts  MaximumApplicationSpeed=60000  SpeedResolution=5e-6  DelayLength=20  MaximumMeasurableSpeed=29999  MeasurableSpeedResolution=1.397e-05  SpeedUnit=Per unit based on dialog  PerUnitSpeed=PU_System.N_base  SpeedDataType=dataType
      settings: SourceProductBaseCode=MT
  speed_PU : Outport
  Pos_PU : Outport  Port=2
  MechPos : Outport  Port=3
  wires:
  IIR Filter4/1 -> speed_PU/1
  Mechanical to Electrical Position/1 -> Pos_PU/1
  Speed Measurement/1 -> IIR Filter4/1
  Quadrature Decoder/1 -> Speed Measurement/1, Calculate Position/1(Theta_m), Mechanical to Electrical Position/1
  Calculate Position/1(Pos) -> MechPos/1
  Encoder Counts/1 -> Quadrature Decoder/1

== system mcb_microchip_pmsm_posCtrl_SAME70/Current Control/Inverter (Simulation)/Subsystem ==
  In1 : Inport
  Constant : Constant  Value=0.5  OutDataTypeStr=dataType
  Gain : Gain  Gain=0.5  OutDataTypeStr=Inherit: Same as input
  Sum : Sum  Inputs=|++
  PWM_Duty_Cycles : Outport
  wires:
  Gain/1 -> Sum/1
  Constant/1 -> Sum/2
  In1/1 -> Gain/1
  Sum/1 -> PWM_Duty_Cycles/1  "PWM_Duty_Cycles"

== system mcb_microchip_pmsm_posCtrl_SAME70/Current Control/Output Scaling/Mode Selector ==
  Delay : Delay  DelayLength=1
  NOT : Logic  Operator=NOT  IconShape=distinctive  AllPortsSameDT=off  OutDataTypeStr=boolean
  Subsystem1 : Subsystem
  Up Counter : Subsystem
  CurrentOffsetEn : Outport
  PosOffset : Outport  Port=2
  wires:
  Up Counter/1(Count) -> Subsystem1/1(Count)
  Delay/1 -> NOT/1
  NOT/1 -> Up Counter/Enable
  Subsystem1/3(EnClosedLoop) -> Delay/1
  Subsystem1/1(Current Offset) -> CurrentOffsetEn/1
  Subsystem1/2(PosOffset) -> PosOffset/1

== system mcb_microchip_pmsm_posCtrl_SAME70/Inverter and Motor/Plant Model/Inverter and Motor (codegen) ==
  Duty_Cycles : Inport
  Ground : Ground
  Terminator : Terminator
  Sim_fb : Outport  VectorParamsAs1DForOutWhenUnconnected=off
  wires:
  Duty_Cycles/1 -> Terminator/1
  Ground/1 -> Sim_fb/1

== system mcb_microchip_pmsm_posCtrl_SAME70/Inverter and Motor/Plant Model/Inverter and Motor (sim) ==
  Duty_Cycles : Inport
  Inverter : Subsystem
  Load_Profile (Torque) : Subsystem
  RT1 : RateTransition  Deterministic=off  OutPortSampleTime=Ts_simulink
  Rate Transition : RateTransition  Deterministic=off  OutPortSampleTime=Ts_motor
  Rate Transition1 : RateTransition  Deterministic=off  OutPortSampleTime=Ts_motor
  Sensor_Measurements : Subsystem
  Surface Mount PMSM : autolibpmsmexterior/Surface Mount PMSM  port_config=Torque  sim_type=Discrete  Ts=Ts_motor  FilePath=surfacepmsm_motordata.m  P=pmsm.p  Rs=pmsm.Rs + inverter.R_board  Ldq_=pmsm.Ld  KConstText=Permanent flux linkage constant (lambda_pm):  lambda_pm=pmsm.FluxPM  Ke=159.9771  Kt=1.323  mechanical=[pmsm.J, pmsm.B, 0]  idq0=[0 0]  theta_init=0  omega_init=0  KConst=pmsm.FluxPM  lambda_pm_calc=pmsm.FluxPM  RefBlkName='autolibpmsmexterior/Surface Mount PMSM'  aMode=5  Ldq="[0.00078136  0.00078136]"
      settings: SourceProductBaseCode=PW,DR,MT,VE
  Terminator : Terminator
  Sim_fb : Outport  VectorParamsAs1DForOutWhenUnconnected=off
  wires:
  Inverter/1(Vabc) -> Rate Transition/1
  Surface Mount PMSM/2 -> RT1/1  "Iabc"
  Sensor_Measurements/1(Sim_fb) -> Sim_fb/1
  Surface Mount PMSM/3 -> Terminator/1
  Load_Profile (Torque)/1(Load_Trq) -> Rate Transition1/1
  Duty_Cycles/1 -> Inverter/1(Duty_abc)
  Rate Transition/1 -> Surface Mount PMSM/2
  Rate Transition1/1 -> Surface Mount PMSM/1
  RT1/1 -> Sensor_Measurements/2(PhaseCurr)
  Surface Mount PMSM/1 -> Sensor_Measurements/1(Info)

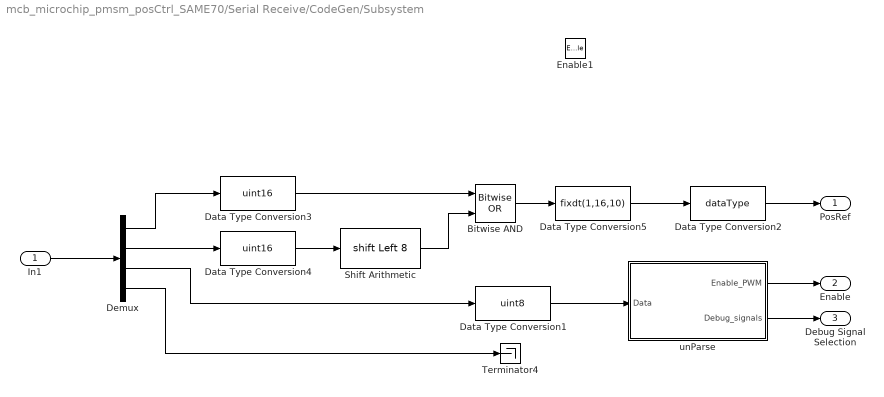
== system mcb_microchip_pmsm_posCtrl_SAME70/Serial Receive/CodeGen/Subsystem ==
  In1 : Inport
  Enable1 : EnablePort
  Bitwise AND : simulink/Logic and Bit Operations/Bitwise Operator  logicop=OR  UseBitMask=off  NumInputPorts=2  BitMask=bin2dec('11011001')  BitMaskRealWorld=Stored Integer
  Data Type Conversion1 : DataTypeConversion  OutDataTypeStr=uint8  RndMeth=Simplest  SaturateOnIntegerOverflow=off
  Data Type Conversion2 : DataTypeConversion  OutDataTypeStr=dataType  RndMeth=Simplest  SaturateOnIntegerOverflow=off
  Data Type Conversion3 : DataTypeConversion  OutDataTypeStr=uint16  RndMeth=Simplest  SaturateOnIntegerOverflow=off
  Data Type Conversion4 : DataTypeConversion  OutDataTypeStr=uint16  RndMeth=Simplest  SaturateOnIntegerOverflow=off
  Data Type Conversion5 : DataTypeConversion  OutDataTypeStr=fixdt(1,16,10)  ConvertRealWorld=Stored Integer (SI)  SaturateOnIntegerOverflow=off
  Demux : Demux
  Shift Arithmetic : ArithShift  BitShiftNumber=8  BitShiftDirection=Left
  Terminator4 : Terminator
  unParse : Subsystem
  PosRef : Outport
  Enable : Outport  Port=2
  Debug Signal Selection : Outport  Port=3
  wires:
  Data Type Conversion4/1 -> Shift Arithmetic/1
  Data Type Conversion3/1 -> Bitwise AND/1
  In1/1 -> Demux/1
  unParse/2(Debug_signals) -> Debug Signal Selection/1
  Data Type Conversion2/1 -> PosRef/1
  Demux/3 -> Data Type Conversion1/1
  Bitwise AND/1 -> Data Type Conversion5/1
  unParse/1(Enable_PWM) -> Enable/1
  Data Type Conversion1/1 -> unParse/1(Data)
  Demux/2 -> Data Type Conversion4/1
  Demux/4 -> Terminator4/1
  Shift Arithmetic/1 -> Bitwise AND/2
  Data Type Conversion5/1 -> Data Type Conversion2/1
  Demux/1 -> Data Type Conversion3/1

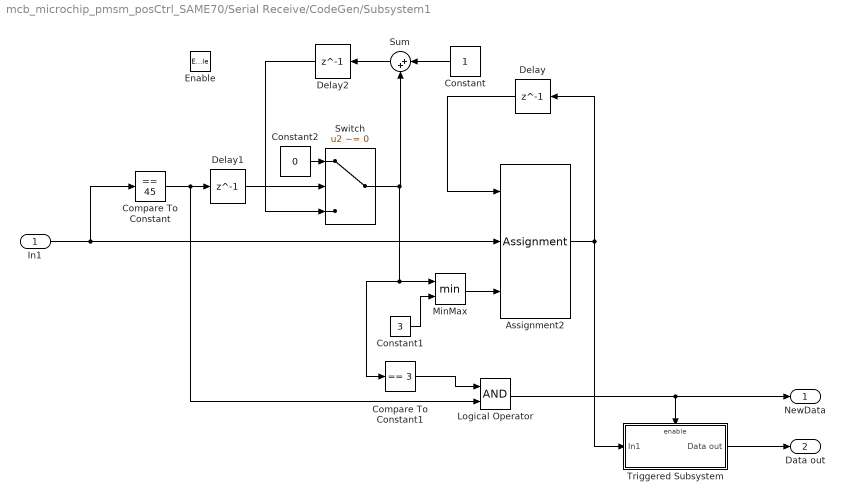
== system mcb_microchip_pmsm_posCtrl_SAME70/Serial Receive/CodeGen/Subsystem1 ==
  In1 : Inport
  Enable : EnablePort
  Assignment2 : Assignment  IndexMode=Zero-based  DiagnosticForDimensions=Warning  IndexOptions=Starting index (port)  Indices=1  OutputSizes=1
  Compare To Constant : simulink/Logic and Bit Operations/Compare To Constant  relop===  const=45  OutDataTypeStr=boolean
  Compare To Constant1 : simulink/Logic and Bit Operations/Compare To Constant  relop===  const=3  OutDataTypeStr=boolean
  Constant : Constant  OutDataTypeStr=uint16  SampleTime=-1
  Constant1 : Constant  Value=3  OutDataTypeStr=uint16  SampleTime=-1
  Constant2 : Constant  Value=0  OutDataTypeStr=uint16  SampleTime=-1
  Delay : Delay  DelayLength=1  InitialCondition=[0 0 0 0]
  Delay1 : Delay  DelayLength=1  InitialCondition=0
  Delay2 : Delay  DelayLength=1  InitialCondition=0
  Logical Operator : Logic  AllPortsSameDT=off  OutDataTypeStr=boolean
  MinMax : MinMax  Inputs=2
  Sum : Sum  Inputs=|++
  Switch : Switch  Criteria=u2 ~= 0  SaturateOnIntegerOverflow=off  InputSameDT=off
  Triggered Subsystem : Subsystem  TreatAsAtomicUnit=on
  NewData : Outport  OutputWhenDisabled=reset  InitialOutput=0
  Data out : Outport  Port=2
  wires:
  Logical Operator/1 -> Triggered Subsystem/Enable, NewData/1
  Triggered Subsystem/1(Data out) -> Data out/1
  Constant2/1 -> Switch/1
  Delay1/1 -> Switch/2
  Switch/1 -> MinMax/1, Compare To Constant1/1, Sum/2
  Sum/1 -> Delay2/1
  MinMax/1 -> Assignment2/3
  Constant1/1 -> MinMax/2
  Constant/1 -> Sum/1
  In1/1 -> Assignment2/2, Compare To Constant/1
  Compare To Constant1/1 -> Logical Operator/1
  Compare To Constant/1 -> Delay1/1, Logical Operator/2
  Delay2/1 -> Switch/3
  Delay/1 -> Assignment2/1
  Assignment2/1 -> Delay/1, Triggered Subsystem/1(In1)

== system mcb_microchip_pmsm_posCtrl_SAME70/Serial Send/Subsystem/Data ==
  Data : Inport
  Action Port : ActionPort  ActionPortLabel=else
  UART Tx : MCHP_Blockset/BUS UART/UART Tx  UART_REF=UART 0  ORDERING=None  AllOrNothing=off  SampleTime=-1  MCHP_MASTERLINK=mcb_microchip_pmsm_posCtrl_SAME70/Configurations/Microchip Master  NSend_Input=off  UART_String=off  NSend_Output=off
      settings: SourceProductName=MPLAB Device Blocks for Simulink
  wires:
  Data/1 -> UART Tx/1

== system mcb_microchip_pmsm_posCtrl_SAME70/Serial Send/Subsystem/End ==
  Data : Inport
  Action Port : ActionPort  ActionPortLabel=elseif(u1 == 119)
  Mux : Mux  Inputs=2
  Start : Constant  Value=hex2dec('45')  OutDataTypeStr=uint8
  UART Tx : MCHP_Blockset/BUS UART/UART Tx  UART_REF=UART 0  ORDERING=None  AllOrNothing=off  SampleTime=-1  MCHP_MASTERLINK=mcb_microchip_pmsm_posCtrl_SAME70/Configurations/Microchip Master  NSend_Input=off  UART_String=off  NSend_Output=off
      settings: SourceProductName=MPLAB Device Blocks for Simulink
  wires:
  Start/1 -> Mux/2
  Data/1 -> Mux/1
  Mux/1 -> UART Tx/1

== system mcb_microchip_pmsm_posCtrl_SAME70/Serial Send/Subsystem/Start ==
  Data : Inport
  Action Port : ActionPort  ActionPortLabel=if(u1 == 0)
  End : Constant  Value=hex2dec('53')  OutDataTypeStr=uint8
  Mux : Mux  Inputs=2
  UART Tx : MCHP_Blockset/BUS UART/UART Tx  UART_REF=UART 0  ORDERING=None  AllOrNothing=off  SampleTime=-1  MCHP_MASTERLINK=mcb_microchip_pmsm_posCtrl_SAME70/Configurations/Microchip Master  NSend_Input=off  UART_String=off  NSend_Output=off
      settings: SourceProductName=MPLAB Device Blocks for Simulink
  wires:
  End/1 -> Mux/1
  Data/1 -> Mux/2
  Mux/1 -> UART Tx/1
